simulink model "PartII_Simulink"  (R2017a)
settings: Solver=ode45  StartTime=0.0  StopTime=0.2  MaxStep=1e-7  RelTol=1e-3
InitFcn:
  | Vg= 7.5;
  | fs = 300e3;
  | 
  | D = 0.44;
  | 
  | R = 26.4;
  | L = 40e-6;
  | C = 0.8e-6;
libraries: powerlib x9, powerlib_meascontrol x1
settings Model: Creator=User  LastModifiedBy=ramiz
settings DataIOCC: SaveFormat=StructureWithTime  ReturnWorkspaceOutputs=on
settings OptimizationCC: LifeSpan=inf
settings DebuggingCC: SFExecutionAtInitializationDiag=none
settings HardwareCC: ProdBitPerSizeT=32  ProdBitPerPtrDiffT=32  ProdWordSize=32  ProdHWDeviceType=Specified
settings SFSimCC: SimUseLocalCustomCode=on
settings RTWCC: RTWUseLocalCustomCode=on

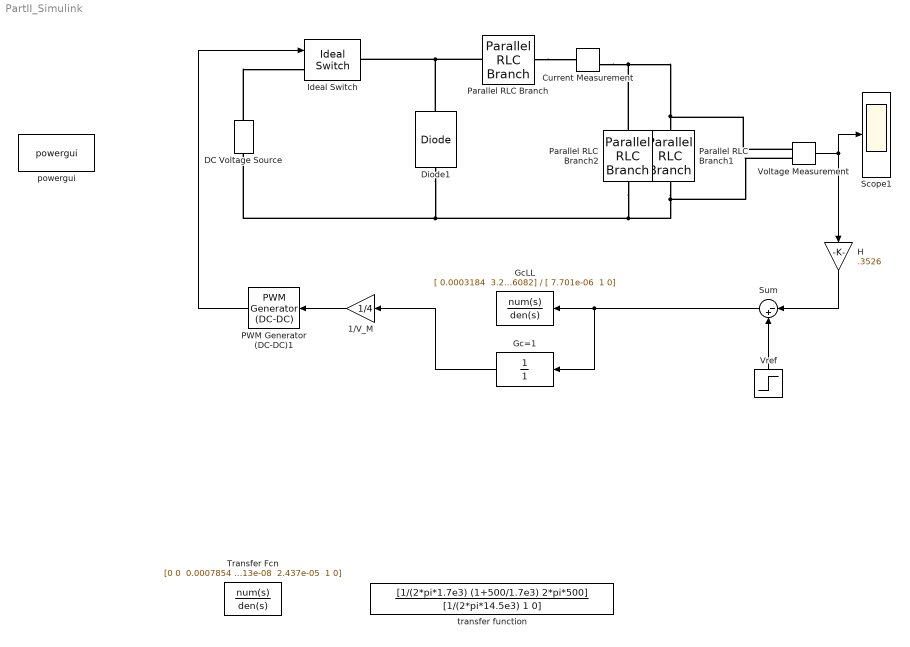
== system PartII_Simulink ==
  1/V_M : Gain  Gain=1/4
  Current Measurement : powerlib/Measurements/Current Measurement  PhasorSimulation=off  OutputType=Complex  PSBequivalent=0
  DC Voltage Source : powerlib/Electrical Sources/DC Voltage Source  Amplitude=28  Measurements=None
  Diode1 : powerlib/Power Electronics/Diode  Ron=1e-6  Lon=0  Vf=0  IC=0  UseSnubber=0  Rs=1e5  Cs=inf  Measurements=off
  Gc=1 : TransferFcn  Denominator=[1]
  GcLL : TransferFcn  Numerator="[ 0.0003184  3.22  6082]"  Denominator="[ 7.701e-06  1 0]"
  H : Gain  Gain=.3526
  Ideal Switch : powerlib/Power Electronics/Ideal Switch  Ron=1e-6  Lon=0  IC=0  Rs=1e9  Cs=inf  Measurements=off
  PWM Generator (DC-DC)1 : powerlib_meascontrol/Pulse & Signal Generators/PWM Generator (DC-DC)  Fsw=100e3  Ts=0
  Parallel RLC Branch : powerlib/Elements/Parallel RLC Branch  LConnTagsString=a  RConnTagsString=__new0  BranchType=L  Resistance=1  Inductance=50e-6  SetiL0=on  InitialCurrent=0  Capacitance=1e-6  Setx0=off  InitialVoltage=0  Measurements=None
  Parallel RLC Branch1 : powerlib/Elements/Parallel RLC Branch  LConnTagsString=a  RConnTagsString=__new0  BranchType=R  Resistance=3  Inductance=1e-3  SetiL0=off  InitialCurrent=0  Capacitance=C  Setx0=on  InitialVoltage=0  Measurements=None
  Parallel RLC Branch2 : powerlib/Elements/Parallel RLC Branch  LConnTagsString=a  RConnTagsString=__new0  BranchType=C  Resistance=R  Inductance=1e-3  SetiL0=off  InitialCurrent=0  Capacitance=500e-6  Setx0=on  InitialVoltage=0  Measurements=None
  Scope1 : Scope
  Sum : Sum  Inputs=|-+
  Transfer Fcn : TransferFcn  Numerator="[0 0  0.0007854  7.943   1.5e04]"  Denominator="[1.925e-13  2.513e-08  2.437e-05  1 0]"
  Voltage Measurement : powerlib/Measurements/Voltage Measurement  PhasorSimulation=off  OutputType=Complex  PSBequivalent=0
  Vref : Step  Time=.05  Before=5.29  After=5.819  SampleTime=0
  powergui : powerlib/powergui  Priority=1  SimulationMode=Discrete  SampleTime=5e-7  frequency=60  Iterations=50  frequencyindice=0  Pbase=100e6  ErrMax=1e-4  UnitsV=kV  UnitsW=MW  buscounter=0  FunctionMessages=off  echomessages=off  EnableUseOfTLC=off  CurrentSourceSwitches=off  DisableSnubberDevices=off  DisableRonSwitches=off  DisableVfSwitches=off  DisplayEquations=off  SolverType=Tustin/Backward Euler (TBE)  Interpol=off  ExternalGateDelay=off  methode=off  Ts=100  x0status=blocks  SPID=on  SwTol=0  HookPort=off  RestoreLinks=warning  ResistiveCurrentMeasurement=off  Frange=[0:2:500]  Ylog=off  Xlog=on  ShowGrid=off  save=off  variable=ZData  structure=output  ZoomFFT=on  StartTime=0.5e-3  cycles=10  DisplayStyle=6  fundamental=300e3  FreqAxis=off  MaxFrequency=3e6  frequencyindicesteady=1  RmsSteady=1  display=off
  transfer function : TransferFcn  Numerator=[1/(2*pi*1.7e3) (1+500/1.7e3) 2*pi*500]  Denominator=[1/(2*pi*14.5e3) 1 0]
  wires:
  Voltage Measurement/1 -> Scope1/1, H/1
  Vref/1 -> Sum/2
  H/1 -> Sum/1
  PWM Generator (DC-DC)1/1 -> Ideal Switch/1
  1/V_M/1 -> PWM Generator (DC-DC)1/1
  Sum/1 -> Gc=1/1, GcLL/1
  Gc=1/1 -> 1/V_M/1
  connections:
  DC Voltage Source/RConn1 -- Ideal Switch/LConn1
  Parallel RLC Branch/LConn1 -- Diode1/RConn1 -- Ideal Switch/RConn1
  Parallel RLC Branch1/RConn1 -- Voltage Measurement/LConn2 -- Parallel RLC Branch2/RConn1 -- DC Voltage Source/LConn1 -- Diode1/LConn1
  Current Measurement/RConn1 -- Parallel RLC Branch2/LConn1 -- Voltage Measurement/LConn1 -- Parallel RLC Branch1/LConn1
  Parallel RLC Branch/RConn1 -- Current Measurement/LConn1
